simulink model "APF_CTL_VIS_Obs_2023a"  (R2023a)
settings: Solver=ode4  StartTime=0.0  StopTime=tsim  FixedStep=baseRate  RelTol=1e-6  AbsTol=1e-6
values from neighbouring files (symbols this model uses):
  A = [0 0 0 1 0 0 ... (first row only)    [CTL_NEW.m]    (also in UKF_SPOT.m = [1 0 0 dt 0 0)
  a = 25.028    [CTL_NEW.m]
  a1 = shape(1)    [Cardioid.m]    (also in Run_Initializer.m = 0.3)
  a2 = shape(2)    [Cardioid.m]    (also in Run_Initializer.m = 0.3)
  a3 = shape(3)    [Cardioid.m]    (also in Run_Initializer.m = 0.4)
  adadelta_epsilon = 1e-5    (= 1e-05)    [Run_Initializer.m]
  adadelta_gamma = 0.37    [Run_Initializer.m]
  adagrad_epsilon = 1e-8    (= 1e-08)    [Run_Initializer.m]
  adagrad_eta = 0.18    [Run_Initializer.m]
  adam_beta_1 = 0.99    [Run_Initializer.m]
  adam_beta_2 = 0.999    [Run_Initializer.m]
  adam_epsilon = 1e-2    (= 0.01)    [Run_Initializer.m]
  adam_eta = 0.0163    [Run_Initializer.m]
  adamax_beta_1 = 0.5    [Run_Initializer.m]
  adamax_beta_2 = 0.999    [Run_Initializer.m]
  adamax_eta = 0.014    [Run_Initializer.m]
  alpha_Black = 0.9    [UKF_SPOT.m]
  alpha_Blue = 0.9    [UKF_SPOT.m]
  Att_Mode = 0    [Run_Initializer.m]
  b1 = shape(4)    [Cardioid.m]    (also in Run_Initializer.m = 0.175)
  b2 = shape(5)    [Cardioid.m]    (also in Run_Initializer.m = 0.175)
  beta_Black = 2    [UKF_SPOT.m]
  beta_Blue = 20    [UKF_SPOT.m]
  Binv = inv(B)    [Run_Initializer.m]
  BLACK_end = [2, 1.4, deg2rad(368)]    [Run_Initializer.m]
  BLACK_ini = [2, 1.4, deg2rad(188), 0, 0, deg2rad(1.5)]    [Run_Initializer.m]
  BLUE_end = [1.3, 1.25, deg2rad(90)]    [Run_Initializer.m]
  BLUE_ini = [1.3, 1.25, deg2rad(270), 0, 0, deg2rad(-1.5)]    [Run_Initializer.m]
  drop_states_BLACK = BLACK_ini(1:3)    [Run_Initializer.m]
  drop_states_BLUE = BLUE_ini(1:3)    [Run_Initializer.m]
  drop_states_RED = RED_ini(1:3)    [Run_Initializer.m]
  dt = 0.01    [UKF_SPOT.m]
  end_time_black = 300    [Run_Initializer.m]
  end_time_blue = 300    [Run_Initializer.m]
  F_max = 0.22    [CTL_NEW.m]
  Gamma1_el = 0.12    [Run_Initializer.m]
  Gamma1_sh = 0.005    [Run_Initializer.m]
  Gamma1_wr = 0.025    [Run_Initializer.m]
  Gamma2_el = 5    [Run_Initializer.m]
  Gamma2_sh = 5    [Run_Initializer.m]
  Gamma2_wr = 5    [Run_Initializer.m]
  Gamma3_el = 10    [Run_Initializer.m]
  Gamma3_sh = 40    [Run_Initializer.m]
  Gamma3_wr = 40    [Run_Initializer.m]
  Gamma4_el = 0.039    [Run_Initializer.m]
  Gamma4_sh = 0.015    [Run_Initializer.m]
  Gamma4_wr = 0.029    [Run_Initializer.m]
  Gamma5_el = 800    [Run_Initializer.m]
  Gamma5_sh = 800    [Run_Initializer.m]
  Gamma5_wr = 800    [Run_Initializer.m]
  Gamma6_el = 0.000001    (= 1e-06)    [Run_Initializer.m]
  Gamma6_sh = 0.005    [Run_Initializer.m]
  Gamma6_wr = 0.02    [Run_Initializer.m]
  H = [1 0 0 0 0 0 ... (first row only)    [UKF_SPOT.m]
  home_states_BLACK = BLACK_ini(1:3)    [Run_Initializer.m]
  home_states_BLUE = BLUE_ini(1:3)    [Run_Initializer.m]
  home_states_RED = RED_ini(1:3)    [Run_Initializer.m]
  Hz = 0.01    [CTL_NEW.m]
  init_states_BLACK = BLACK_ini(1:3)    [Run_Initializer.m]
  init_states_BLUE = BLUE_ini(1:3)    [Run_Initializer.m]
  init_states_RED = RED_ini(1:3)    [Run_Initializer.m]
  J = IRED    [CTL_NEW.m]    (also in UKF_SPOT.m = 0.20184)
  k = lqr(A,B1,Q,R)    [CTL_NEW.m]
  k_1_0 = k(1,1)    [CTL_NEW.m]
  k_1_t_0 = k(3,3)    [CTL_NEW.m]
  k_2_0 = k(1,4)    [CTL_NEW.m]
  k_2_t_0 = k(3,6)    [CTL_NEW.m]
  K_a = diag([2 2 3.5])    [Run_Initializer.m]
  ka = 1    [Run_Initializer.m]
  Kd_elarm = 0.8    [Run_Initializer.m]
  Kd_sharm = 1.0    (= 1)    [Run_Initializer.m]
  Kd_t = 9.5    [CTL_NEW.m]    (also in Run_Initializer.m)
  Kd_wrarm = 0.6    [Run_Initializer.m]
  Kd_x = 28    [CTL_NEW.m]    (also in Run_Initializer.m)
  Kd_y = Kd_x    (= 28)    [CTL_NEW.m]    (also in Run_Initializer.m)
  Kp_elarm = 1.2    [Run_Initializer.m]
  Kp_sharm = 1.5    [Run_Initializer.m]
  Kp_t = 1    [CTL_NEW.m]    (also in Run_Initializer.m)
  Kp_wrarm = 2    [Run_Initializer.m]
  Kp_x = 3.5    [CTL_NEW.m]    (also in Run_Initializer.m)
  Kp_y = Kp_x    (= 3.5)    [CTL_NEW.m]    (also in Run_Initializer.m)
  kr = 2    [Run_Initializer.m]
  lambda1 = 0.4    [CTL_NEW.m]
  lambda12 = 0.4    [CTL_NEW.m]
  lambda12_t = 0.05    [CTL_NEW.m]
  lambda1_t = 0.05    [CTL_NEW.m]
  lambda2 = 0.4    [CTL_NEW.m]
  lambda2_t = 0.05    [CTL_NEW.m]
  lamda_Black = (alpha_Black^2)*(N + kappa_Black) - N    (= 15.06)    [UKF_SPOT.m]
  lamda_Blue = (alpha_Blue^2)*(N + kappa_Blue) - N    (= 6.96)    [UKF_SPOT.m]
  m = mRED    [CTL_NEW.m]    (also in UKF_SPOT.m = 11.21)
  method = 1    [UKF_SPOT.m]
  Method = 8    [Run_Initializer.m]
  momentum_eta = 0.7    [Run_Initializer.m]
  momentum_gamma = 0.7    [Run_Initializer.m]
  nesterov_eta = 0.6    [Run_Initializer.m]
  nesterov_gamma = 0.3    [Run_Initializer.m]
  Nmat = diag([1 1 1])    [Run_Initializer.m]
  p = 0.4    [CTL_NEW.m]
  P_b = diag([45 45 0])    [Run_Initializer.m]
  P_IC_Black = 0.2*eye(6)    [UKF_SPOT.m]
  P_IC_Blue = 0.2*eye(6)    [UKF_SPOT.m]
  p_t = 0.05    [CTL_NEW.m]
  psi = 1    [Run_Initializer.m]
  PWMFreq = 5    [Run_Initializer.m]
  Q = [w 0 0 0 0 0 ... (first row only)    [CTL_NEW.m]
  Q_a = diag([5, 5, 0])    [Run_Initializer.m]
  Q_b = diag([0.0125, 0.0125, 0.05])    [Run_Initializer.m]
  Q_Black = [0.0000005 0 0 0 0 0 ... (first row only)    [UKF_SPOT.m]
  Q_Blue = [0.000075 0 0 0 0 0 ... (first row only)    [UKF_SPOT.m]
  R = [r 0 0 ... (first row only)    [CTL_NEW.m]
  R_Black = [variance 0 0 ... (first row only)    [UKF_SPOT.m]
  R_Blue = [variance 0 0 ... (first row only)    [UKF_SPOT.m]
  r_hold = 0.427    [Run_Initializer.m]
  r_off = 0.165    [Run_Initializer.m]
  RED_ini = [2.7, 0.4, deg2rad(135+360), 0, 0, 0]    [Run_Initializer.m]
  Red_Rate = 0.025    [CTL_NEW.m]
  RMSprop_epsilon = 1e-8    (= 1e-08)    [Run_Initializer.m]
  RMSprop_eta = 0.025    [Run_Initializer.m]
  RMSprop_gamma = 0.9    [Run_Initializer.m]
  ... (+11 more)
undefined symbols (not defined in the file or in its folder): alpha, alpha_m, alphap, alphat, Am, b, b0, b3, baseRate, beta, Bm, c, Cm, d, DiscIntNeverNeededParam, Dm, drop_states_ARM, epsilon, F_Black_X_nominal, F_Black_Y_nominal, F_Blue_X_nominal, F_Blue_Y_nominal, F_red_X_nominal, F_red_Y_nominal, F_thrusters_BLACK, F_thrusters_BLUE, F_thrusters_RED, IBLACK, IBLUE, IDIST, IEE, IPROX, IRED, K, k1, k1t, k2, k2t, K_t, Kd_tb, Kd_tblue, Kd_tr, Kd_xb, Kd_xblue, Kd_xr, Kd_yb, Kd_yblue, Kd_yr, Kp_tb, Kp_tblue, Kp_tr, Kp_xb, Kp_xblue, Kp_xr, Kp_yb, Kp_yblue, Kp_yr, lamda ... (+34)
libraries: nvidiaSharedBlocks x10, MainLibrary x4, dspsigops x4, simulink x2, etargetslib x1
(part 13 of 15)

== matlab function APF_CTL_VIS_Obs_2023a/Phase #3: Experiment/Change RED Behavior/Sub-Phase #4/BLACK/UKF_New/MATLAB Function2 ==
  data: no_IC output; States output; P_K output; Reject_Sum output; Reject output; Measurments input; Force input; States_k1 input; P_K1 input; lamda_Black parameter; J parameter; m parameter; dt parameter; Q_Black parameter; alpha_Black parameter; beta_Black parameter; H parameter; R_Black parameter; thresh_Black parameter; method parameter; Reject_sumk1 input; Reject_k1 input; thresh_Factor_Black parameter
function [no_IC,States,P_K,Reject_Sum,Reject] = UKF(Measurments,Force,States_k1,P_K1, lamda_Black, J, m, dt, Q_Black, alpha_Black, beta_Black, H, R_Black,thresh_Black, method,Reject_sumk1,Reject_k1, thresh_Factor_Black)
%% Block diagram got messy so i put it all in one block
if isempty(Force)
    Force = [0;0;0];
end

%% Inital position
if all(States_k1 == 0) || anynan(States_k1)
    if anynan(Measurments)
        States = NaN(6,1);
        no_IC = 1;
        P_K = P_K1;
        Reject_Sum = 0;
        Reject = 0;
    else
        States = [Measurments;zeros(3,1)];
        no_IC = 0;
        P_K = P_K1;
        Reject_Sum = 0;
        Reject = 0;
    end
else
    no_IC = 0;

    X_Cal = fcn1(States_k1,P_K1,lamda_Black,method);
    
    X_Cal_k1 = fcn2(Force,X_Cal,J,m,dt);
    
    [w_m,w_c,X_tilda_k,P_K1] = fcn3(X_Cal_k1,lamda_Black, Q_Black, alpha_Black, beta_Black);
    
    [Z_Bar,Z_Cal] = fcn4(X_Cal_k1, w_m,H);
    
    [P_xz_k,P_z_k] = fcn5(Z_Bar,Z_Cal,w_c,X_tilda_k,X_Cal,R_Black);
    
    K_k = fcn6(P_xz_k,P_z_k);
    
    Z_k = fcn7(Measurments);

    [thresh_Dynamic,Reject_Sum] = Dyn_Thresh(thresh_Black,Reject_k1,thresh_Factor_Black,Reject_sumk1);
    
    Reject = fcn8(Z_k,Z_Bar,P_z_k,thresh_Dynamic);
    
    States = fcn9(Z_k,Reject,X_tilda_k,Z_Bar,K_k);
    
    P_K = fcn10(P_K1,P_z_k,K_k,Reject);
end
end

function X_Cal = fcn1(x_tilda_k,P_k,lamda,method)
%% Calculate size of sigma var
sz = 6;
N = 2*sz + 1;
X_Cal = zeros(sz,N);

%% Calculate initial sigma point
X_Cal(:,1) = x_tilda_k;

%% Calculate sigma distance
sigma = (6 + lamda)*P_k;
sigma = Cholesky_Decomposition(sigma,method);

%% Calculate Sigma Points
% Positive points
for i = 2:1:((N-1)/2) + 1
    fill = zeros(size(x_tilda_k));
    fill(i-1,1) = sigma(i-1,i-1);
    X_Cal(:,i) = x_tilda_k + fill;
end
% Negative Points
j = 1;
for i = N + 1 - ((N-1)/2):1:N
    fill = zeros(size(x_tilda_k));
    fill(j,1) = sigma(j,j);
    X_Cal(:,i) = x_tilda_k - fill;
    j = j + 1;
end
end

function L = Cholesky_Decomposition(mat,method)

%% Getting size of matrix
[row,col] = size(mat);

%% Make sure matrix can be decomposed
if ~isequal(size(mat), size(mat'))
    error('Input matrix must be symmetric');
end

if any(eig(mat) <= 0)
    % error('Input matrix must be positive definite'); %% Added Error
    % Handling
    mat = NearPositiveDefinite(mat,method);
end

%% Pre allocating Space
L = zeros(row,col);

% Perform Cholesky decomposition
    for i = 1:col
        % Compute the diagonal element
        L(i, i) = sqrt(mat(i, i) - sum(L(i, 1:i-1).^2));
        
        % Compute the elements below the diagonal
        for j = i+1:col
            L(j, i) = (mat(j, i) - sum(L(j, 1:i-1).*L(i, 1:i-1))) / L(i, i);
        end
    end
end

function A_P = NearPositiveDefinite(A,method)
%% Method 1 (Symmetric Polar Factor)
%% Method 2 (Eigenvalue Recomposition)
    % enforce symmetry
    if isreal(A)
        B = 0.5*(A + A');
    else
        B = 0.5*(A + A');
        B = real(B) + 1i*hermSign(B).*imag(B);
    end

    if method == 1
        [~,~,U] = svd(B);
        H = U*U';
        A = (B + H)/2;

    elseif method == 2
        % Eigenvalue recomposition with modification for complex matrices
        [V,D] = eig(B);
        if isreal(A)
            D = max(real(D), 0); % Ensure real part of eigenvalues is non-negative
        else
            % For complex matrices, ensure positive semidefinite
            D = max(D, 0); % Ensure eigenvalues are non-negative
            V = real(V); % Take the real part of eigenvectors
        end
        A = real(V)*real(D)*real(V)'; % Now this really real product really should be really real right?
    else
        error('Please select proper method for Near Positive Definite Iteration')
    end

    % enforce symmetry again
    A_P = 0.5*(A + A');

    % Iteration
    i = 1;
    j = 0;
    max_iterations = 1000; % Maximum iterations allowed before increment starts increasing exponentially
    large_j_threshold = 500; % Threshold value for j to start increasing increment exponentially

    while i ~= 0
        [~,i] = chol(A_P);
        j = j + 1;
        if i ~= 0 % if close, add a multiple of the identity scaled by the smallest eigenvalue
            eig_min = min(eig(A_P));
            if j <= large_j_threshold
                increment = (-real(eig_min)*j.^2 + eps(real(eig_min)))*eye(size(A));
            else
                % Increase increment exponentially
                increment = (abs(real(eig_min))*j.^2 + eps(real(eig_min)))*exp(0.1*(j - large_j_threshold))*eye(size(A));
            end
            A_P = A_P + increment;
        end
        if j > max_iterations % If j exceeds the maximum allowed iterations, break the loop
            break;
        end
    end
end

function X_Cal_k1  = fcn2( F, X_Cal_k, J, m, dt)
%% Pre-Define
X_Cal_k1 = zeros(size(X_Cal_k));
%% System Dynamics
A = [eye(3), eye(3)*dt;
    zeros(3), eye(3)];

B = [eye(2)*(dt^2)/(2*m), zeros(2,1);
     0,0, (dt^2)/(2*J);
     eye(2)*(dt)/(m), zeros(2,1);
     0,0, (dt)/(J)];

%% State propigation
f = size(X_Cal_k,2);
for i = 1:1:f
    X_Cal_k1(:,i) = A*X_Cal_k(:,i) + B*F; 
end
end

function [w_m,w_c,X_tilda_k,P_K] = fcn3(X_Cal_k1,lamda, Q, alpha, beta)
%% Sigma weights
sz = size(X_Cal_k1,2);
N = 6;

%% For non modifyed variation
% w_0 = kappa/(N + kappa);
% w_i = 1/(2*(N + kappa));
% w = w_i*ones(1,N);
% w(1,1) = w_0;

%% Additional step - Sigma Points Weights
w_m_0 = lamda/(N + lamda);
w_c_0 = (lamda/(N + lamda)) + beta + (1 - alpha^2);
w_i = 1/(2*(N + lamda));

w = w_i*ones(1,sz-1);
w_m = [w_m_0, w];
w_c = [w_c_0, w];

w_m = diag(w_m);
w_c = diag(w_c);

%% State Prediction
X_tilda_k = X_Cal_k1*w_m;
X_tilda_k = sum(X_tilda_k,2);


%% Covariance Prediction
P_K = (X_Cal_k1 - X_tilda_k)*w_c*(X_Cal_k1 - X_tilda_k)' + Q;

end

function [Z_Bar,Z_Cal] = fcn4(x_Cal_k1, w_m,H)
%% calc Z_Cal
N = size(x_Cal_k1,2);
Z_Cal = zeros(3,N);
for i = 1:1:N
    Z_Cal(:,i) = H*x_Cal_k1(:,i);
end

%% Calc Z_Bar
Z_Bar = Z_Cal*w_m;
Z_Bar = sum(Z_Bar,2);
end

function [P_xz_k,P_z_k] = fcn5(Z_Bar,Z_Cal,w_c,x_tilda_k1,X_Cal,R)
%% calc P_z
P_z_k = (Z_Cal - Z_Bar)*w_c*(Z_Cal - Z_Bar)' + R;

%% calc P_xz
P_xz_k = (X_Cal - x_tilda_k1)*w_c*(Z_Cal - Z_Bar)';
end

function K_k = fcn6(P_xz_k,P_z_k)
K_k = (P_xz_k)*P_z_k';
end

function Z_k = fcn7(z_k)
    %% Assuming that all states are given or no states are given
    if anynan(z_k)
        Z_k = 1000*ones(3,1);
    else
    Z_k = z_k;
    end
end

function  Reject = fcn8(Z_k,Z_Bar,P_z_k,thresh)
%% Calc Mahalanobis Distance
D_square = (transpose(Z_k - Z_Bar))*P_z_k*(Z_k - Z_Bar);
% mahalanobis_d = sqrt(D_square);

%% Determine if data should be rejected
if D_square < thresh
    Reject = 0;
else
    Reject = 1;
end
end

function [x] = fcn9(z,Reject,X_tilda_k,z_bar,K_k)
%% State estimate
    if Reject == 0
        x = X_tilda_k + K_k*(z - z_bar);
    else
        x = X_tilda_k;
    end
end

function P_K = fcn10(P_k1,P_z_k,K_k,Reject)
if Reject == 0
    P_K = P_k1 - (K_k*P_z_k)*K_k';
else
    P_K = P_k1;
end
end


function [thresh_Dynamic,Reject_Sum] = Dyn_Thresh(thresh_Black,Reject_k1,thresh_Factor_Black,Reject_sumk1)
if Reject_k1 == 1    
    Reject_Sum = Reject_sumk1 + 1;
    thresh_Dynamic = thresh_Black + Reject_Sum*thresh_Factor_Black;
else 
    Reject_Sum = 0;
    thresh_Dynamic = thresh_Black;
end
end

== matlab function APF_CTL_VIS_Obs_2023a/Phase #3: Experiment/Change RED Behavior/Sub-Phase #4/BLACK/MATLAB Function3 ==
  data: Measurments input; Black_Measurments_table_ref output; Red_States input
function Black_Measurments_table_ref = RelitivetoTable(Measurments,Red_States)
 Measurments(1) = Measurments(1)/100;
 Measurments(2) = Measurments(2)/100;
 Measurments(3) = Measurments(3)*pi/180;

%% This code is very scuffed, so I added lots of notes, feel free to change this
%% Size check
if size(Red_States,1) == 6 || size(Red_States,2) == 6
    Red_States = Red_States(1:3);
elseif size(Red_States,1) == 3 || size(Red_States,2) == 3
    % Nothin
else
    disp('Error with demensions of Red_States')
    disp('Please use 3 or 6 states')
    disp(':(')
end

if size(Measurments,1) == 3 || size(Measurments,2) == 3
    % Nothin
else
    disp('Error with demensions of Measurments')
    disp('VIS only gives 3 states, please only use 3 states')
    disp(':(')
end

%% Rotation matrix scuffed (accounts for the location change of the docking cone)
    c3 = [sin(Red_States(3)),  cos(Red_States(3)), 0;
          cos(Red_States(3)), -sin(Red_States(3)), 0;
          0,                     0,                    1];

%% Measurments in table ref frame
    Black_Measurments_table_ref = c3*Measurments;

%% Vector addition
    Black_Measurments_table_ref(1) = Black_Measurments_table_ref(1) + Red_States(1); 
    Black_Measurments_table_ref(2) =  -1*Black_Measurments_table_ref(2) + Red_States(2); % Negative Y value accounting for "Left Hand Rule"

%% Angle addition
    Black_Measurments_table_ref(3) = Measurments(3) + Red_States(3) - pi/2; % Pi/2 for the docking cone location offset from Phase Space

%% Wrapping Angle from -pi to pi
% Dont ask me why, its consistant with the SPOT inport from phasespace
% Dont belive me, look at this, angular velocity is being unwrapped, therefor, angle must be wrapped
% APF_Path_Planning_2023a/PhaseSpace Camera Code/Use Hardware to Obtain States
    Black_Measurments_table_ref(3) = mod(Black_Measurments_table_ref(3) + pi, 2*pi) - pi;
end

== matlab function APF_CTL_VIS_Obs_2023a/Phase #5: Hold Home/Change BLUE Behavior/Hough Control/MATLAB Function2 ==
  data: Oy output; z input; Ox output
function [Oy, Ox]   = C3( z )
%C3 gives the rotation matrix about the z-axis for an angle 'z'
%   z - the angle about the z-axis which you rotate
%   A - the rotation matrix

Ox = [cos(z) sin(z); -sin(z) cos(z)]*[1;0];
Oy = [cos(z) sin(z); -sin(z) cos(z)]*[0;1];
end

== matlab function APF_CTL_VIS_Obs_2023a/Phase #3: Experiment/Change RED Behavior/Sub-Phase #4/GDC/Target Tracker/Constant Angular Rate/Looking Angle ==
  data: state_black input; state_red input; theta_desired output; r_off parameter
function theta_desired = fcn(state_black, state_red, r_off)

p_l = [state_black(1) + r_off*cos(state_black(3));
       state_black(2) + r_off*sin(state_black(3))];

p_c_1 = state_red(1:2);
r_cl = p_c_1 - p_l;

r_cl_x = r_cl(1);
r_cl_y = r_cl(2);

theta_desired = angle(r_cl_x + 1j*r_cl_y) + pi;

== matlab function APF_CTL_VIS_Obs_2023a/Phase #3: Experiment/Change RED Behavior/Sub-Phase #4/CTL/Target Finder/LQR1/MATLAB Function ==
  data: k input; u output; q1_x input; q2_x input; q1_y input; q2_y input; q1_t input; q2_t input
function u = fcn(k,q1_x,q2_x,q1_y,q2_y,q1_t,q2_t)

x = [q1_x;
    q1_y;
    q1_t;
    q2_x;
    q2_y;
    q2_t];

u = k*x;
% u = [0; 0; 0];

== matlab function APF_CTL_VIS_Obs_2023a/Phase #3: Experiment/Change BLUE Behavior/Sub-Phase #2 /MATLAB Function2 ==
  data: t input; x output; xLength parameter
function x = fcn(t, xLength)

x = -0.85*cos((0.03490659)*t) + xLength/2;

end

== matlab function APF_CTL_VIS_Obs_2023a/Phase #3: Experiment/Change BLUE Behavior/Sub-Phase #2 /MATLAB Function3 ==
  data: t input; y output; yLength parameter
function y = fcn(t, yLength)

y = -0.85*sin((0.03490659)*t) + yLength/2;

end

== matlab function APF_CTL_VIS_Obs_2023a/Phase #3: Experiment/Change RED Behavior/Sub-Phase #4/BLACK/MEKF/MATLAB Function ==
  data: Measurments input; States output; F input; X_tilda_k input; P_k1 input; P_K output; J parameter; m parameter; dt parameter; Q parameter; R parameter; H parameter; thresh parameter
function [States, P_K]  = MEKF(Measurments,F,X_tilda_k,P_k1, J, m, dt, Q, R, H, thresh)

if isempty(F)
    F = [0;0;0];
end

    %% Body
    [x_tilda_k1,P_k1] = fcn1( F, m, J, dt, X_tilda_k, P_k1,Q);
    
    K_k = fcn2(P_k1,R, H);

    Z_k = fcn7(Measurments);
    
    Y_k = fcn3(Z_k,H,x_tilda_k1);
    
    [~, Reject] = fnc4(Z_k, x_tilda_k1, P_k1,thresh,H);
    
    States = fcn5(Y_k,X_tilda_k,Reject,K_k);
    
    P_K = fcn(P_k1,K_k,H);
end

function [x_tilda_k1,P_k1] = fcn1( F, m, J, dt, X_tilda_k, P_k,Q)

A = [eye(3), eye(3)*dt;
    zeros(3), eye(3)];

G = [eye(2)*(dt^2)/(2*m), zeros(2,4);
     zeros(1,2), (dt^2)/(2*J), zeros(1,3);
     zeros(2,4), eye(2)*(dt)/(m);
     zeros(1,5), (dt)/(J)];
B = [eye(2)*(dt^2)/(2*m), zeros(2,1);
     0,0, (dt^2)/(2*J);
     eye(2)*(dt)/(m),zeros(2,1);
     0,0, (dt)/(J)];

x_tilda_k1 = A*X_tilda_k + B*F; %State prediction
P_k1 = A'*P_k*A;
P_k1 = P_k1 + G'*Q*G; %covariance predict
P_k1 = 0.5*(P_k1 + P_k1'); %enforce symmetric
end

function K_k = fcn2(P_k1,R, H)
Sk = H*P_k1*H' + R;
K_k = P_k1*H'*inv(Sk);
end

function Z_k = fcn7(z_k)
    %% Assuming that all states are given or no states are given
    if anynan(z_k)
        Z_k = 1000*ones(3,1);
    else
    Z_k = z_k;
    end
end

function Y_k = fcn3(Z_k,H,X_tilda_k1)
Y_k = Z_k - H*X_tilda_k1;
end

function [mahalanobis_d, Reject] = fnc4(z_k, X_tilda_k1, Pk1,thresh,H)
    % measurement: Measurement vector
    % stateEstimate: Estimated state vector (6x1)
    % covarianceMatrix: Covariance matrix of the state estimate (6x6)

    % Number of state variables
    numVariables = length(X_tilda_k1);

    % Residual vector
    residual = z_k - H*X_tilda_k1;

    % Mahalanobis distance calculation
    mahalanobis_d = sqrt(residual' * inv(Pk1(1:3,1:3)) * residual);
    threshold = thresh;

    % If Mahalanobis distance exceeds the threshold, consider it an outlier
    if mahalanobis_d > threshold
        Reject = 1;
    else
        Reject = 0;
    end
end

function x = fcn5(Y_k,X_tilda_k,Reject,K_k)
    if Reject == 0
        x = X_tilda_k + K_k*Y_k;
    else
        x = X_tilda_k;
    end
end

function P_K = fcn(P_k1,K_k,H)
P_K = zeros(6,6);
P_K = (eye(6) - K_k*H)*P_k1*transpose(eye(6) - K_k*H) + K_k*K_k'; 
P_k = 0.5*(P_K'+P_K); % make covariance matrix symmetric
end

== matlab function APF_CTL_VIS_Obs_2023a/Thruster Control Code/Change BLUE Behavior/Calculate Thruster ON//OFF/MATLAB Function6 ==
  data: thrust_decay_factor output; PWMs input; thruster_count_threshold parameter; count output
function [thrust_decay_factor, count]  = check_thrust_decay(PWMs,thruster_count_threshold)

% normalize PWMs
if max(PWMs) > 1
    PWMs = PWMs/max(PWMs);
end

count = sum(PWMs > thruster_count_threshold);

positives_only = max(PWMs,0);
sum_of_duty_cycles = sum(positives_only);

average_duty_cycle_per_thruster = sum_of_duty_cycles/count;

% Look up the thrust decay for this average duty cycle
if (average_duty_cycle_per_thruster < 0.3) || (count == 0)
    thrust_decay_factor = 1;
else
    thrust_decay_factor = max(0.6 - 2*average_duty_cycle_per_thruster + 1, 0.5);   
end

== matlab function APF_CTL_VIS_Obs_2023a/Thruster Control Code/Change BLUE Behavior/Calculate Thruster ON//OFF/MATLAB Function7 ==
  data: H output; thruster_dist2CG_BLUE parameter; F_Blue_X_nominal parameter; thrust_decay_factor input; F_Blue_Y_nominal parameter
function H   = MakeHWithDecay(thruster_dist2CG_BLUE,F_Blue_X_nominal, thrust_decay_factor, F_Blue_Y_nominal)


adjusted_thruster_dist2CG_BLUE = [thruster_dist2CG_BLUE(1);
                                 thruster_dist2CG_BLUE(2);
                                 thruster_dist2CG_BLUE(3);
                                 thruster_dist2CG_BLUE(4);
                                 thruster_dist2CG_BLUE(5);
                                 thruster_dist2CG_BLUE(6);
                                 thruster_dist2CG_BLUE(7);
                                 thruster_dist2CG_BLUE(8)];
                                 


Vec1 = [ -1
         -1
          0 
          0
          1
          1
          0
          0 ];
      
Vec2 = [  0
          0
          1
          1
          0
          0
         -1
         -1 ];
     
Vec3 = adjusted_thruster_dist2CG_BLUE./1000;

Mat1 = [Vec1, Vec2, Vec3]';

F_thrusters_BLUE = [F_Blue_X_nominal*thrust_decay_factor; F_Blue_X_nominal*thrust_decay_factor; F_Blue_Y_nominal*thrust_decay_factor; F_Blue_Y_nominal*thrust_decay_factor; F_Blue_X_nominal*thrust_decay_factor; F_Blue_X_nominal*thrust_decay_factor; F_Blue_Y_nominal*thrust_decay_factor; F_Blue_Y_nominal*thrust_decay_factor];

Mat2 = diag((F_thrusters_BLUE./2));

H    = Mat1*Mat2;

end

== matlab function APF_CTL_VIS_Obs_2023a/Phase #5: Hold Home/Change BLUE Behavior/Hough Control/MATLAB Function3 ==
  data: z input; Ox output
function Ox    = C3( z )
%C3 gives the rotation matrix about the z-axis for an angle 'z'
%   z - the angle about the z-axis which you rotate
%   A - the rotation matrix

Ox = [cos(z) sin(z); -sin(z) cos(z)]*[1;0];
end

== matlab function APF_CTL_VIS_Obs_2023a/Thruster Control Code/Change BLACK Behavior/Calculate Thruster ON//OFF/MATLAB Function10 ==
  data: thrust_decay_factor output; PWMs input; thruster_count_threshold parameter; count output
function [thrust_decay_factor, count]  = check_thrust_decay(PWMs,thruster_count_threshold)

% normalize PWMs
if max(PWMs) > 1
    PWMs = PWMs/max(PWMs);
end

count = sum(PWMs > thruster_count_threshold);

positives_only = max(PWMs,0);
sum_of_duty_cycles = sum(positives_only);

average_duty_cycle_per_thruster = sum_of_duty_cycles/count;

% Look up the thrust decay for this average duty cycle
if (average_duty_cycle_per_thruster < 0.3) || (count == 0)
    thrust_decay_factor = 1;
else
    thrust_decay_factor = max(0.6 - 2*average_duty_cycle_per_thruster + 1, 0.5);   
end

== matlab function APF_CTL_VIS_Obs_2023a/Thruster Control Code/Change BLACK Behavior/Calculate Thruster ON//OFF/MATLAB Function11 ==
  data: H output; thruster_dist2CG_BLACK parameter; F_Black_X_nominal parameter; thrust_decay_factor input; F_Black_Y_nominal parameter
function H   = MakeHWithDecay(thruster_dist2CG_BLACK,F_Black_X_nominal, thrust_decay_factor, F_Black_Y_nominal)


adjusted_thruster_dist2CG_BLACK = [thruster_dist2CG_BLACK(1);
                                 thruster_dist2CG_BLACK(2);
                                 thruster_dist2CG_BLACK(3);
                                 thruster_dist2CG_BLACK(4);
                                 thruster_dist2CG_BLACK(5);
                                 thruster_dist2CG_BLACK(6);
                                 thruster_dist2CG_BLACK(7);
                                 thruster_dist2CG_BLACK(8)];
                                 


Vec1 = [ -1
         -1
          0 
          0
          1
          1
          0
          0 ];
      
Vec2 = [  0
          0
          1
          1
          0
          0
         -1
         -1 ];
     
Vec3 = adjusted_thruster_dist2CG_BLACK./1000;

Mat1 = [Vec1, Vec2, Vec3]';

F_thrusters_BLACK = [F_Black_X_nominal*thrust_decay_factor; F_Black_X_nominal*thrust_decay_factor; F_Black_Y_nominal*thrust_decay_factor; F_Black_Y_nominal*thrust_decay_factor; F_Black_X_nominal*thrust_decay_factor; F_Black_X_nominal*thrust_decay_factor; F_Black_Y_nominal*thrust_decay_factor; F_Black_Y_nominal*thrust_decay_factor];

Mat2 = diag((F_thrusters_BLACK./2));

H    = Mat1*Mat2;

end

== matlab function APF_CTL_VIS_Obs_2023a/Phase #3: Experiment/Change RED Behavior/Sub-Phase #4/BLACK/UKF1/MATLAB Function ==
  data: Measurments input; States output; Force input; States_k1 input; P_K1 input; P_K output; lamda parameter; J parameter; m parameter; dt parameter; Q parameter; alpha parameter; beta parameter; H parameter; R parameter; thresh parameter
function [States,P_K] = UKF(Measurments,Force,States_k1,P_K1, lamda, J, m, dt, Q, alpha, beta, H, R, thresh)
%% Block diagram got messy so i put it all in one block
if isempty(Force)
    Force = [0;0;0];
end

X_Cal= fcn1(States_k1,P_K1,lamda);

X_Cal_k1 = fcn2(Force,X_Cal,J,m,dt);

[w_m,w_c,X_tilda_k,P_K1] = fcn3(X_Cal_k1,lamda, Q, alpha, beta);

[Z_Bar,Z_Cal] = fcn4(X_Cal_k1, w_m,H);

[P_xz_k,P_z_k] = fcn5(Z_Bar,Z_Cal,w_c,X_tilda_k,X_Cal,R);

K_k = fcn6(P_xz_k,P_z_k);

Z_k = fcn7(Measurments);

Reject = fcn8(Z_k,Z_Bar,P_z_k,thresh);

States = fcn9(Z_k,Reject,X_tilda_k,Z_Bar,K_k);

P_K = fcn10(P_K1,P_z_k,K_k,Reject);
end

function X_Cal = fcn1(x_tilda_k,P_k,lamda)
%% Calculate size of sigma var
sz = 6;
N = 2*sz + 1;
X_Cal = zeros(sz,N);

%% Calculate initial sigma point
X_Cal(:,1) = x_tilda_k;

%% Calculate sigma distance
sigma = (6 + lamda)*P_k;
sigma = Cholesky_Decomposition(sigma);

%% Calculate Sigma Points
% Positive points
for i = 2:1:((N-1)/2) + 1
    fill = zeros(size(x_tilda_k));
    fill(i-1,1) = sigma(i-1,i-1);
    X_Cal(:,i) = x_tilda_k + fill;
end
% Negative Points
j = 1;
for i = N + 1 - ((N-1)/2):1:N
    fill = zeros(size(x_tilda_k));
    fill(j,1) = sigma(j,j);
    X_Cal(:,i) = x_tilda_k - fill;
    j = j + 1;
end
end

function L = Cholesky_Decomposition(mat)
%% Getting size of matrix
[row,col] = size(mat);
%% Make sure matrix can be decomposed
if row ~= col
    disp('Error due to matrix size')
    disp('Make sure square matrix is input into Cholesky Decoposition')
end

if ~isequal(size(mat), size(mat'))
    error('Input matrix must be symmetric');
end

if any(eig(mat) <= 0)
    error('Input matrix must be positive definite');
end

%% Pre allocating Space
L = zeros(row,col);

% Perform Cholesky decomposition
    for i = 1:col
        % Compute the diagonal element
        L(i, i) = sqrt(mat(i, i) - sum(L(i, 1:i-1).^2));
        
        % Compute the elements below the diagonal
        for j = i+1:col
            L(j, i) = (mat(j, i) - sum(L(j, 1:i-1).*L(i, 1:i-1))) / L(i, i);
        end
    end
end

function X_Cal_k1  = fcn2( F, X_Cal_k, J, m, dt)
%% Pre-Define
X_Cal_k1 = zeros(size(X_Cal_k));
%% System Dynamics
A = [eye(3), eye(3)*dt;
    zeros(3), eye(3)];

B = [eye(2)*(dt^2)/(2*m), zeros(2,1);
     0,0, (dt^2)/(2*J);
     eye(2)*(dt)/(m), zeros(2,1);
     0,0, (dt)/(J)];

%% State propigation
f = size(X_Cal_k,2);
for i = 1:1:f
    X_Cal_k1(:,i) = A*X_Cal_k(:,i) + B*F; 
end
end

function [w_m,w_c,X_tilda_k,P_K] = fcn3(X_Cal_k1,lamda, Q, alpha, beta)
%% Sigma weights
sz = size(X_Cal_k1,2);
N = 6;

%% For non modifyed variation
% w_0 = kappa/(N + kappa);
% w_i = 1/(2*(N + kappa));
% w = w_i*ones(1,N);
% w(1,1) = w_0;

%% Additional step - Sigma Points Weights
w_m_0 = lamda/(N + lamda);
w_c_0 = (lamda/(N + lamda)) + beta + (1 - alpha^2);
w_i = 1/(2*(N + lamda));

w = w_i*ones(1,sz-1);
w_m = [w_m_0, w];
w_c = [w_c_0, w];

w_m = diag(w_m);
w_c = diag(w_c);

%% State Prediction
X_tilda_k = X_Cal_k1*w_m;
X_tilda_k = sum(X_tilda_k,2);


%% Covariance Prediction
P_K = (X_Cal_k1 - X_tilda_k)*w_c*(X_Cal_k1 - X_tilda_k)' + Q;

end

function [Z_Bar,Z_Cal] = fcn4(x_Cal_k1, w_m,H)
%% calc Z_Cal
N = size(x_Cal_k1,2);
Z_Cal = zeros(3,N);
for i = 1:1:N
    Z_Cal(:,i) = H*x_Cal_k1(:,i);
end

%% Calc Z_Bar
Z_Bar = Z_Cal*w_m;
Z_Bar = sum(Z_Bar,2);
end

function [P_xz_k,P_z_k] = fcn5(Z_Bar,Z_Cal,w_c,x_tilda_k1,X_Cal,R)
%% calc P_z
P_z_k = (Z_Cal - Z_Bar)*w_c*(Z_Cal - Z_Bar)' + R;

%% calc P_xz
P_xz_k = (X_Cal - x_tilda_k1)*w_c*(Z_Cal - Z_Bar)';
end

function K_k = fcn6(P_xz_k,P_z_k)
K_k = (P_xz_k)*P_z_k';
end

function Z_k = fcn7(z_k)
    %% Assuming that all states are given or no states are given
    if anynan(z_k)
        Z_k = 1000*ones(3,1);
    else
    Z_k = z_k;
    end
end

function  Reject = fcn8(Z_k,Z_Bar,P_z_k,thresh)
%% Calc Mahalanobis Distance
D_square = (transpose(Z_k - Z_Bar))*P_z_k*(Z_k - Z_Bar);
% mahalanobis_d = sqrt(D_square);

%% Determine if data should be rejected
if D_square < thresh
    Reject = 0;
else
    Reject = 1;
end
end

function [x] = fcn9(z,Reject,X_tilda_k,z_bar,K_k)
%% State estimate
    if Reject == 0
        x = X_tilda_k + K_k*(z - z_bar);
    else
        x = X_tilda_k;
    end
end

function P_K = fcn10(P_k1,P_z_k,K_k,Reject)
if Reject == 0
    P_K = P_k1 - (K_k*P_z_k)*K_k';
else
    P_K = P_k1;
end
end

== matlab function APF_CTL_VIS_Obs_2023a/Phase #3: Experiment/Change BLUE Behavior/Sub-Phase #3 /Hough Control/MATLAB Function2 ==
  data: Oy output; z input; Ox output
function [Oy, Ox]   = C3( z )
%C3 gives the rotation matrix about the z-axis for an angle 'z'
%   z - the angle about the z-axis which you rotate
%   A - the rotation matrix

Ox = [cos(z) sin(z); -sin(z) cos(z)]*[1;0];
Oy = [cos(z) sin(z); -sin(z) cos(z)]*[0;1];
end

== matlab function APF_CTL_VIS_Obs_2023a/Phase #3: Experiment/Change BLUE Behavior/Sub-Phase #3 /Hough Control/MATLAB Function3 ==
  data: z input; Ox output
function Ox    = C3( z )
%C3 gives the rotation matrix about the z-axis for an angle 'z'
%   z - the angle about the z-axis which you rotate
%   A - the rotation matrix

Ox = [cos(z) sin(z); -sin(z) cos(z)]*[1;0];
end

== matlab function APF_CTL_VIS_Obs_2023a/Phase #3: Experiment/Change BLUE Behavior/Sub-Phase #3 /Hough Control/MATLAB Function4 ==
  data: Oy input; e_out output; e_in input
function e_out = fcn(Oy, e_in)

a = sign(Oy'*e_in);
e_out = -a*norm(e_in);

== matlab function APF_CTL_VIS_Obs_2023a/Phase #3: Experiment/Change BLUE Behavior/Sub-Phase #3 /MATLAB Function2 ==
  data: t input; x output; xLength parameter
function x = fcn(t, xLength)

x = -0.85*cos((0.03490659)*t) + xLength/2;

end

== matlab function APF_CTL_VIS_Obs_2023a/Phase #5: Hold Home/Change BLUE Behavior/Hough Control/MATLAB Function4 ==
  data: Oy input; e_out output; e_in input
function e_out = fcn(Oy, e_in)

a = sign(Oy'*e_in);
e_out = -a*norm(e_in);

== matlab function APF_CTL_VIS_Obs_2023a/Phase #3: Experiment/Change BLUE Behavior/Sub-Phase #3 /MATLAB Function3 ==
  data: t input; y output; yLength parameter
function y = fcn(t, yLength)

y = -0.85*sin((0.03490659)*t) + yLength/2;

end

== matlab function APF_CTL_VIS_Obs_2023a/Phase #3: Experiment/Change RED Behavior/Sub-Phase #4/BLACK/Parker's Transform ==
  data: rel_state_black input; state_red input; abs_state_black output
function abs_state_black = fcn(rel_state_black,state_red)
%calcualtes ECI pos/att of black

% messing with rel state black
rel_state_black(1) = rel_state_black(1)/100;
rel_state_black(2) = rel_state_black(2)/100;
rel_state_black(3) = rel_state_black(3)*(pi/180)+pi/2; 

angle = -state_red(3);

C = [cos(angle),sin(angle);
     -sin(angle),cos(angle)];

abs_distance_black = C*[rel_state_black(1);rel_state_black(2)];

abs_pos_black = [state_red(1);state_red(2)] + abs_distance_black;

abs_angle_black = rel_state_black(3) - state_red(3);

abs_state_black =  [abs_pos_black;
                    abs_angle_black];

== matlab function APF_CTL_VIS_Obs_2023a/Phase #3: Experiment/Change RED Behavior/Sub-Phase #4/BLACK/Kalman Filter1/MATLAB Function ==
  data: z_k input; Z_k output
function Z_k = fcn(z_k)
    %% Assuming that all states are given or no states are given
    if anynan(z_k)
        Z_k = zeros(3,1);
    else
    Z_k = z_k;
    end
end

== matlab function APF_CTL_VIS_Obs_2023a/Phase #3: Experiment/Change RED Behavior/Sub-Phase #4/BLACK/Kalman Filter1/MATLAB Function1 ==
  data: P_k input; P_k1 output; A parameter; Q_T parameter
function P_k1 = fcn(P_k,A, Q_T)
if isempty(P_k) 
    P_k1 = Peye(6);
else
    P_k1 = A*P_k*(transpose(A)) + Q_T;
end
end

== matlab function APF_CTL_VIS_Obs_2023a/Phase #3: Experiment/Change RED Behavior/Sub-Phase #4/BLACK/Kalman Filter1/MATLAB Function2 ==
  data: P_k1 input; K_k output; H parameter; R parameter
function K_k = fcn(P_k1,H, R)

K_k = P_k1*(transpose(H))/(H*P_k1*(transpose(H)) + R);
end

== matlab function APF_CTL_VIS_Obs_2023a/Phase #3: Experiment/Change RED Behavior/Sub-Phase #4/BLACK/Kalman Filter1/MATLAB Function3 ==
  data: P_k1 input; P_K output; K_k input; H parameter
function P_K = fcn(P_k1,K_k,H)
P_K = zeros(6,6);
P_K = P_k1 - (K_k*H*P_k1); 
end

== matlab function APF_CTL_VIS_Obs_2023a/Phase #3: Experiment/Change RED Behavior/Sub-Phase #4/BLACK/Kalman Filter1/MATLAB Function4 ==
  data: Z_k input; x output; X_tilda_k input; K_k input; H parameter
function x = fcn(Z_k,X_tilda_k,K_k,H)

x = X_tilda_k + K_k*(Z_k - H*X_tilda_k);
end

== matlab function APF_CTL_VIS_Obs_2023a/Phase #3: Experiment/Change RED Behavior/Sub-Phase #4/BLACK/Kalman Filter1/MATLAB Function5 ==
  data: X_tilda_k1 input; x_tilda_k output; A parameter
function x_tilda_k = fcn(X_tilda_k1,A)

x_tilda_k = A*X_tilda_k1;
end

== matlab function APF_CTL_VIS_Obs_2023a/Phase #3: Experiment/Change RED Behavior/Sub-Phase #4/CTL/Target Tracker/LQR1/MATLAB Function ==
  data: k input; u output; q1_x input; q2_x input; q1_y input; q2_y input; q1_t input; q2_t input
function u = fcn(k,q1_x,q2_x,q1_y,q2_y,q1_t,q2_t)

x = [q1_x;
    q1_y;
    q1_t;
    q2_x;
    q2_y;
    q2_t];

u = k*x;
% u = [0; 0; 0];

== matlab function APF_CTL_VIS_Obs_2023a/Phase #5: Hold Home/Change RED Behavior/Hough Control/MATLAB Function2 ==
  data: Oy output; z input; Ox output
function [Oy, Ox]   = C3( z )
%C3 gives the rotation matrix about the z-axis for an angle 'z'
%   z - the angle about the z-axis which you rotate
%   A - the rotation matrix

Ox = [cos(z) sin(z); -sin(z) cos(z)]*[1;0];
Oy = [cos(z) sin(z); -sin(z) cos(z)]*[0;1];
end

== matlab function APF_CTL_VIS_Obs_2023a/Phase #3: Experiment/Change RED Behavior/Sub-Phase #4/CTL/If Action Subsystem/CSMC3/MATLAB Function ==
  data: phi input; u output; alphap parameter
function u = fcn(phi, alphap)



u = sign(phi)*(abs(phi)^(alphap/(2 - alphap)));

== matlab function APF_CTL_VIS_Obs_2023a/Phase #3: Experiment/Change RED Behavior/Sub-Phase #4/GDC/Target Finder/Constant Angular Rate/Wrap1/MATLAB Function ==
  data: u input; wrappedAngle output
function wrappedAngle = wrapAngle(u)

wrappedAngle = atan2(sin(u),cos(u));

end

== matlab function APF_CTL_VIS_Obs_2023a/Phase #3: Experiment/Change RED Behavior/Sub-Phase #4/CTL/If Action Subsystem/CSMC3/MATLAB Function1 ==
  data: q2 input; u output; k1 parameter; alphap parameter
function u = fcn(q2,k1, alphap)

u = sign(k1*q2)*(abs(k1*q2)^alphap);

== matlab function APF_CTL_VIS_Obs_2023a/Phase #3: Experiment/Change RED Behavior/Sub-Phase #4/CTL/If Action Subsystem/CSMC3/MATLAB Function2 ==
  data: q1 input; phi output; k1 parameter; alphap parameter; q2 input
function phi = fcn(q1,k1, alphap, q2)



phi = k1*q1 + (1/(2 - alphap))*sign(k1*q2)*(abs(k1*q2))^(2 - alphap);

== matlab function APF_CTL_VIS_Obs_2023a/Phase #3: Experiment/Change RED Behavior/Sub-Phase #4/CTL/If Action Subsystem/CSMC3/MATLAB Function3 ==
  data: phi input; u output; alphap parameter
function u = fcn(phi, alphap)



u = sign(phi)*(abs(phi)^(alphap/(2 - alphap)));

== matlab function APF_CTL_VIS_Obs_2023a/Phase #3: Experiment/Change RED Behavior/Sub-Phase #4/CTL/If Action Subsystem/CSMC3/MATLAB Function4 ==
  data: q2 input; u output; k1 parameter; alphap parameter
function u = fcn(q2,k1, alphap)

u = sign(k1*q2)*(abs(k1*q2)^alphap);

== matlab function APF_CTL_VIS_Obs_2023a/Phase #3: Experiment/Change RED Behavior/Sub-Phase #4/CTL/If Action Subsystem/CSMC3/MATLAB Function5 ==
  data: q1 input; phi output; k1 parameter; alphap parameter; q2 input
function phi = fcn(q1,k1, alphap, q2)



phi = k1*q1 + (1/(2 - alphap))*sign(k1*q2)*(abs(k1*q2))^(2 - alphap);

== matlab function APF_CTL_VIS_Obs_2023a/Phase #3: Experiment/Change RED Behavior/Sub-Phase #4/CTL/If Action Subsystem/CSMC3/MATLAB Function6 ==
  data: phi input; u output; alpha parameter
function u = fcn(phi, alpha)



u = sign(phi)*(abs(phi)^(alpha/(2 - alpha)));

== matlab function APF_CTL_VIS_Obs_2023a/Phase #3: Experiment/Change RED Behavior/Sub-Phase #4/CTL/If Action Subsystem/CSMC3/MATLAB Function7 ==
  data: q2 input; u output; k1 parameter; alpha parameter
function u = fcn(q2,k1, alpha)

u = sign(k1*q2)*(abs(k1*q2)^alpha);

== matlab function APF_CTL_VIS_Obs_2023a/Phase #5: Hold Home/Change RED Behavior/Hough Control/MATLAB Function3 ==
  data: z input; Ox output
function Ox    = C3( z )
%C3 gives the rotation matrix about the z-axis for an angle 'z'
%   z - the angle about the z-axis which you rotate
%   A - the rotation matrix

Ox = [cos(z) sin(z); -sin(z) cos(z)]*[1;0];
end

== matlab function APF_CTL_VIS_Obs_2023a/Phase #3: Experiment/Change RED Behavior/Sub-Phase #4/CTL/If Action Subsystem/CSMC3/MATLAB Function8 ==
  data: q1 input; phi output; k1 parameter; alpha parameter; q2 input
function phi = fcn(q1,k1, alpha, q2)



phi = k1*q1 + (1/(2 - alpha))*sign(k1*q2)*(abs(k1*q2))^(2 - alpha);

== matlab function APF_CTL_VIS_Obs_2023a/Phase #3: Experiment/Change RED Behavior/Sub-Phase #4/CTL/If Action Subsystem/DAC Controller2/Fx Gain Derivatives ==
  data: e_xdot input; k2_dot output; e_x input; k1_dot output; lambda1 parameter; lambda2 parameter; lambda12 parameter; p parameter
function [k2_dot, k1_dot]= fcn(e_xdot, e_x, lambda1, lambda2, lambda12, p)

k1_dot = -lambda1*p*e_x^2-(lambda1+p*lambda12)*e_x*e_xdot-lambda12*e_xdot^2;
k2_dot = -lambda12*p*e_x^2-(lambda12+p*lambda2)*e_x*e_xdot-lambda2*e_xdot^2;

== matlab function APF_CTL_VIS_Obs_2023a/Phase #3: Experiment/Change RED Behavior/Sub-Phase #4/CTL/If Action Subsystem/DAC Controller2/Fy Gain Derivatives ==
  data: k2_dot output; e_ydot input; e_y input; k1_dot output; lambda1 parameter; lambda2 parameter; lambda12 parameter; p parameter
function [k2_dot, k1_dot]= fcn(e_ydot, e_y, lambda1, lambda2, lambda12, p)

k1_dot = -lambda1*p*e_y^2-(lambda1+p*lambda12)*e_y*e_ydot-lambda12*e_ydot^2;
k2_dot = -lambda12*p*e_y^2-(lambda12+p*lambda2)*e_y*e_ydot-lambda2*e_ydot^2;

== matlab function APF_CTL_VIS_Obs_2023a/Phase #3: Experiment/Change RED Behavior/Sub-Phase #4/CTL/If Action Subsystem/DAC Controller2/Torque Gain Derivatives ==
  data: e_t input; e_tdot input; k1_dot output size=1; k2_dot output size=1; lambda1_t parameter; lambda2_t parameter; lambda12_t parameter; p_t parameter
function [k1_dot, k2_dot]= fcn(e_t, e_tdot, lambda1_t, lambda2_t, lambda12_t, p_t)
k1_dot = -lambda1_t*p_t*e_t^2-(lambda1_t+p_t*lambda12_t)*e_t*e_tdot-lambda12_t*e_tdot^2;
k2_dot = -lambda12_t*p_t*e_t^2-(lambda12_t+p_t*lambda2_t)*e_t*e_tdot-lambda2_t*e_tdot^2;

== matlab function APF_CTL_VIS_Obs_2023a/Phase #3: Experiment/Change RED Behavior/Sub-Phase #4/CTL/If Action Subsystem/Homo/MATLAB Function ==
  data: q1 input; u output; k1 parameter; alphap parameter
function u = fcn(q1,k1, alphap)

u = k1*sign(q1)*(abs(q1)^(alphap/(2 - alphap)));

== matlab function APF_CTL_VIS_Obs_2023a/Phase #3: Experiment/Change RED Behavior/Sub-Phase #4/CTL/If Action Subsystem/Homo/MATLAB Function1 ==
  data: q2 input; u output; k2 parameter; alphap parameter
function u = fcn(q2,k2, alphap)

u = k2*sign(q2)*(abs(q2)^alphap);

== matlab function APF_CTL_VIS_Obs_2023a/Phase #3: Experiment/Change RED Behavior/Sub-Phase #4/CTL/If Action Subsystem/DAC Controller1/Fy Gain Derivatives ==
  data: k2_dot output; e_ydot input; e_y input; k1_dot output; lambda1 parameter; lambda2 parameter; lambda12 parameter; p parameter
function [k2_dot, k1_dot]= fcn(e_ydot, e_y, lambda1, lambda2, lambda12, p)

k1_dot = -lambda1*p*e_y^2-(lambda1+p*lambda12)*e_y*e_ydot-lambda12*e_ydot^2;
k2_dot = -lambda12*p*e_y^2-(lambda12+p*lambda2)*e_y*e_ydot-lambda2*e_ydot^2;

== matlab function APF_CTL_VIS_Obs_2023a/Phase #5: Hold Home/Change RED Behavior/Hough Control/MATLAB Function4 ==
  data: Oy input; e_out output; e_in input
function e_out = fcn(Oy, e_in)

a = sign(Oy'*e_in);
e_out = -a*norm(e_in);

== matlab function APF_CTL_VIS_Obs_2023a/Phase #3: Experiment/Change RED Behavior/Sub-Phase #4/CTL/If Action Subsystem/DAC Controller1/Torque Gain Derivatives ==
  data: e_t input; e_tdot input; k1_dot output size=1; k2_dot output size=1; lambda1_t parameter; lambda2_t parameter; lambda12_t parameter; p_t parameter
function [k1_dot, k2_dot]= fcn(e_t, e_tdot, lambda1_t, lambda2_t, lambda12_t, p_t)
k1_dot = -lambda1_t*p_t*e_t^2-(lambda1_t+p_t*lambda12_t)*e_t*e_tdot-lambda12_t*e_tdot^2;
k2_dot = -lambda12_t*p_t*e_t^2-(lambda12_t+p_t*lambda2_t)*e_t*e_tdot-lambda2_t*e_tdot^2;

== matlab function APF_CTL_VIS_Obs_2023a/Phase #3: Experiment/Change RED Behavior/Sub-Phase #4/CTL/If Action Subsystem/Homo/MATLAB Function4 ==
  data: q1 input; u output; k1t parameter; alphat parameter
function u = fcn(q1,k1t, alphat)

u = k1t*sign(q1)*(abs(q1)^(alphat/(2 - alphat)));

== matlab function APF_CTL_VIS_Obs_2023a/Phase #3: Experiment/Change RED Behavior/Sub-Phase #4/CTL/If Action Subsystem/Homo/MATLAB Function5 ==
  data: q2 input; u output; k2t parameter; alphat parameter
function u = fcn(q2,k2t, alphat)

u = k2t*sign(q2)*(abs(q2)^alphat);

== matlab function APF_CTL_VIS_Obs_2023a/Phase #3: Experiment/Change RED Behavior/Sub-Phase #4/CTL/If Action Subsystem/LQR/MATLAB Function ==
  data: k input; u output; q1_x input; q2_x input; q1_y input; q2_y input; q1_t input; q2_t input
function u = fcn(k,q1_x,q2_x,q1_y,q2_y,q1_t,q2_t)

x = [q1_x;
    q1_y;
    q1_t;
    q2_x;
    q2_y;
    q2_t];

u = k*x;
% u = [0; 0; 0];

== matlab function APF_CTL_VIS_Obs_2023a/Phase #3: Experiment/Change RED Behavior/Sub-Phase #4/CTL/If Action Subsystem/Sat/MATLAB Function ==
  data: q2 input; q1 input; saturation output; a1 parameter; b parameter; m parameter
function saturation = fcn(q2,q1,a1, b, m)

u = a1*m*q1 + a1*m*q2/b;

saturation = u;

== matlab function APF_CTL_VIS_Obs_2023a/Phase #3: Experiment/Change RED Behavior/Sub-Phase #4/CTL/If Action Subsystem/Sat/MATLAB Function1 ==
  data: q2 input; q1 input; saturation output; a1 parameter; b parameter; m parameter
function saturation = fcn(q2,q1,a1, b, m)

u = a1*m*q1 + a1*m*q2/b;

saturation = u;

== matlab function APF_CTL_VIS_Obs_2023a/Phase #3: Experiment/Change RED Behavior/Sub-Phase #4/CTL/If Action Subsystem/Sat/MATLAB Function2 ==
  data: q2 input; q1 input; saturation output; c parameter; d parameter; J parameter
function saturation = fcn(q2,q1,c, d, J)

u = c*J*q1 + c*J*q2/d;

saturation = u;

== matlab function APF_CTL_VIS_Obs_2023a/Simulate Plant Dynamics/RED and ARM Dynamics/RED + ARM/RED + ARM Dynamics/Coriolis Function1 ==
  data: a1 parameter; a2 parameter; a3 parameter; b0 parameter; b1 parameter; b2 parameter; mPROX parameter; mDIST parameter; mEE parameter; Phi parameter; CoriolisS output; x input
function CoriolisS = CoriolisFunc3LINK(a1,a2,a3,b0,b1,b2,mPROX,mDIST,mEE,Phi,x)
%CORIOLISFUNC3LINK
%    CORIOLISS = CORIOLISFUNC3LINK(A1,A2,A3,B0,B1,B2,mPROX,mDIST,mEE,PHI,Q0,Q1,Q2,Q3,Q0_DOT,Q1_DOT,Q2_DOT,Q3_DOT)

%    This function was generated by the Symbolic Math Toolbox version 8.0.
%    05-Nov-2017 11:48:44

q0 = x(3);
q1 = x(4);
q2 = x(5);
q3 = x(6);

q0_dot = x(9);
q1_dot = x(10);
q2_dot = x(11);
q3_dot = x(12);

t2 = a1+b1;
t3 = a1.*mPROX;
t4 = mDIST.*t2;
t5 = mEE.*t2;
t6 = t3+t4+t5;
t7 = a2.*mDIST;
t8 = a2+b2;
t9 = mEE.*t8;
t10 = t7+t9;
t11 = pi.*(1.0./2.0);
t12 = q0_dot.*t6;
t13 = q1_dot.*t6;
t14 = q0+q1+t11;
t15 = cos(t14);
t16 = t12+t13;
t17 = q0_dot.*t10;
t18 = q1_dot.*t10;
t19 = q2_dot.*t10;
t20 = q0+q1+q2+t11;
t21 = cos(t20);
t22 = t17+t18+t19;
t23 = a3.*mEE.*q0_dot;
t24 = a3.*mEE.*q1_dot;
t25 = a3.*mEE.*q2_dot;
t26 = a3.*mEE.*q3_dot;
t27 = q0+q1+q2+q3+t11;
t28 = cos(t27);
t29 = t23+t24+t25+t26;
t30 = b0.*mPROX;
t31 = b0.*mDIST;
t32 = b0.*mEE;
t33 = t30+t31+t32;
t34 = (pi/2-Phi)+q0;
t35 = sin(t14);
t36 = sin(t20);
t37 = sin(t27);
t38 = q0_dot+q1_dot+q2_dot+q3_dot;
t39 = q0+q1+q2+q3;
t40 = a1.*b0.*mPROX.*q1_dot;
t41 = a1.*b0.*mDIST.*q1_dot;
t42 = a1.*b0.*mEE.*q1_dot;
t43 = b0.*b1.*mDIST.*q1_dot;
t44 = b0.*b1.*mEE.*q1_dot;
t45 = (pi/2-Phi)-q1;
t46 = cos(t45);
t47 = a2.*b0.*mDIST.*q1_dot;
t48 = a2.*b0.*mDIST.*q2_dot;
t49 = a2.*b0.*mEE.*q1_dot;
t50 = a2.*b0.*mEE.*q2_dot;
t51 = b0.*b2.*mEE.*q1_dot;
t52 = b0.*b2.*mEE.*q2_dot;
t53 = -(pi/2-Phi)+q1+q2;
t54 = cos(t53);
t55 = a3.*b0.*mEE.*q1_dot;
t56 = a3.*b0.*mEE.*q2_dot;
t57 = a3.*b0.*mEE.*q3_dot;
t58 = -(pi/2-Phi)+q1+q2+q3;
t59 = cos(t58);
t60 = a2.*b1.*mDIST.*q2_dot;
t61 = a1.*b2.*mEE.*q2_dot;
t62 = a2.*b1.*mEE.*q2_dot;
t63 = b1.*b2.*mEE.*q2_dot;
t64 = a1.*a2.*mDIST.*q2_dot;
t65 = a1.*a2.*mEE.*q2_dot;
t66 = sin(q2);
t67 = t60+t61+t62+t63+t64+t65;
t68 = a3.*b2.*mEE.*q3_dot;
t69 = a2.*a3.*mEE.*q3_dot;
t70 = sin(q3);
t71 = t68+t69;
t72 = a3.*b1.*mEE.*q2_dot;
t73 = a3.*b1.*mEE.*q3_dot;
t74 = a1.*a3.*mEE.*q2_dot;
t75 = a1.*a3.*mEE.*q3_dot;
t76 = q2+q3;
t77 = sin(t76);
t78 = t72+t73+t74+t75;
t79 = a2.*b0.*mDIST.*q0_dot;
t80 = a2.*b0.*mEE.*q0_dot;
t81 = b0.*b2.*mEE.*q0_dot;
t82 = t47+t48+t49+t50+t51+t52+t79+t80+t81;
t83 = a3.*b0.*mEE.*q0_dot;
t84 = t55+t56+t57+t83;
t85 = a1.*b0.*mPROX.*q0_dot;
t86 = a1.*b0.*mDIST.*q0_dot;
t87 = a1.*b0.*mEE.*q0_dot;
t88 = b0.*b1.*mDIST.*q0_dot;
t89 = b0.*b1.*mEE.*q0_dot;
t90 = a2.*b1.*mDIST.*q0_dot;
t91 = a1.*b2.*mEE.*q0_dot;
t92 = a2.*b1.*mDIST.*q1_dot;
t93 = a2.*b1.*mEE.*q0_dot;
t94 = a1.*b2.*mEE.*q1_dot;
t95 = a2.*b1.*mEE.*q1_dot;
t96 = b1.*b2.*mEE.*q0_dot;
t97 = b1.*b2.*mEE.*q1_dot;
t98 = a1.*a2.*mDIST.*q0_dot;
t99 = a1.*a2.*mDIST.*q1_dot;
t100 = a1.*a2.*mEE.*q0_dot;
t101 = a1.*a2.*mEE.*q1_dot;
t102 = t60+t61+t62+t63+t64+t65+t90+t91+t92+t93+t94+t95+t96+t97+t98+t99+t100+t101;
t103 = a3.*b1.*mEE.*q0_dot;
t104 = a3.*b1.*mEE.*q1_dot;
t105 = a1.*a3.*mEE.*q0_dot;
t106 = a1.*a3.*mEE.*q1_dot;
t107 = t72+t73+t74+t75+t103+t104+t105+t106;
t108 = t79+t80+t81;
t109 = t54.*t108;
t110 = t59.*t83;
t111 = t90+t91+t92+t93+t94+t95+t96+t97+t98+t99+t100+t101;
t112 = t66.*t111;
t113 = t103+t104+t105+t106;
t114 = t77.*t113;
t115 = a2.*q0_dot;
t116 = a2.*q1_dot;
t117 = a2.*q2_dot;
t118 = b2.*q0_dot;
t119 = b2.*q1_dot;
t120 = b2.*q2_dot;
t121 = t115+t116+t117+t118+t119+t120;
t122 = a3.*mEE.*t70.*t121;
t123 = a1.*q0_dot;
t124 = a1.*q1_dot;
t125 = b1.*q0_dot;
t126 = b1.*q1_dot;
t127 = t123+t124+t125+t126;
t128 = a3.*mEE.*t77.*t127;
CoriolisS = reshape([0.0,0.0,0.0,0.0,0.0,0.0,0.0,0.0,0.0,0.0,0.0,0.0,-t15.*t16-t21.*t22-t28.*t29-q0_dot.*t33.*cos(t34),-t16.*t35-t22.*t36-t29.*t37-q0_dot.*t33.*sin(t34),-t66.*t67-t70.*t71-t77.*t78-t46.*(t40+t41+t42+t43+t44)-t59.*(t55+t56+t57)-t54.*(t47+t48+t49+t50+t51+t52),t109+t110-t66.*t67-t70.*t71-t77.*t78+t46.*(t85+t86+t87+t88+t89),t109+t110+t112+t114-t70.*t71,t110+t122+t128,-t15.*t16-t21.*t22-t28.*t29,-t16.*t35-t22.*t36-t29.*t37,-t66.*t67-t54.*t82-t70.*t71-t59.*t84-t77.*t78-t46.*(t40+t41+t42+t43+t44+t85+t86+t87+t88+t89),-t66.*t67-t70.*t71-t77.*t78,t112+t114-t70.*t71,t122+t128,-t21.*t22-t28.*t29,-t22.*t36-t29.*t37,-t54.*t82-t70.*t71-t59.*t84-t66.*t102-t77.*t107,-t70.*t71-t66.*t102-t77.*t107,-a3.*mEE.*q3_dot.*t8.*t70,a3.*mEE.*t8.*t70.*(q0_dot+q1_dot+q2_dot),a3.*mEE.*t38.*sin(t39),-a3.*mEE.*t38.*cos(t39),-a3.*b0.*mEE.*t38.*t59-a3.*mEE.*t8.*t38.*t70-a3.*mEE.*t2.*t38.*t77,-a3.*mEE.*t8.*t38.*t70-a3.*mEE.*t2.*t38.*t77,-a3.*mEE.*t8.*t38.*t70,0.0],[6,6]);
end

== matlab function APF_CTL_VIS_Obs_2023a/Phase #3: Experiment/Change RED Behavior/Sub-Phase #4/CTL/If Action Subsystem/Sat/MATLAB Function3 ==
  data: q2 input; u input; saturation output; F_max parameter; e parameter; b parameter; m parameter
function saturation = fcn(q2,u,F_max, e, b, m)

if u >= e
    u = e;
elseif u <= -1*e
    u = -1*e;
else
    u = u;
end

u = b*q2*m + u;

if u >= F_max
    u = F_max;
elseif u <= -1*F_max
    u = -1*F_max;
else
    u = u;
end

saturation = u;
